simulink subsystem "wheelSlip"  (R2022b)
settings: Solver=VariableStepAuto  StartTime=0.0  StopTime=10.0  RelTol=1e-3
libraries: wheels x3
settings Model: Creator=serga  LastModifiedBy=serga

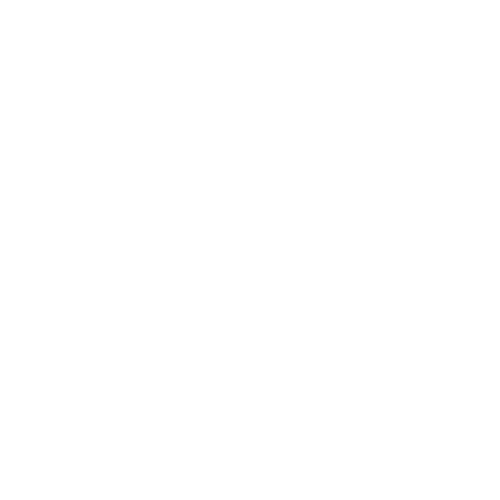
[thumbnail: Simulink's stored preview of the top-level diagram]
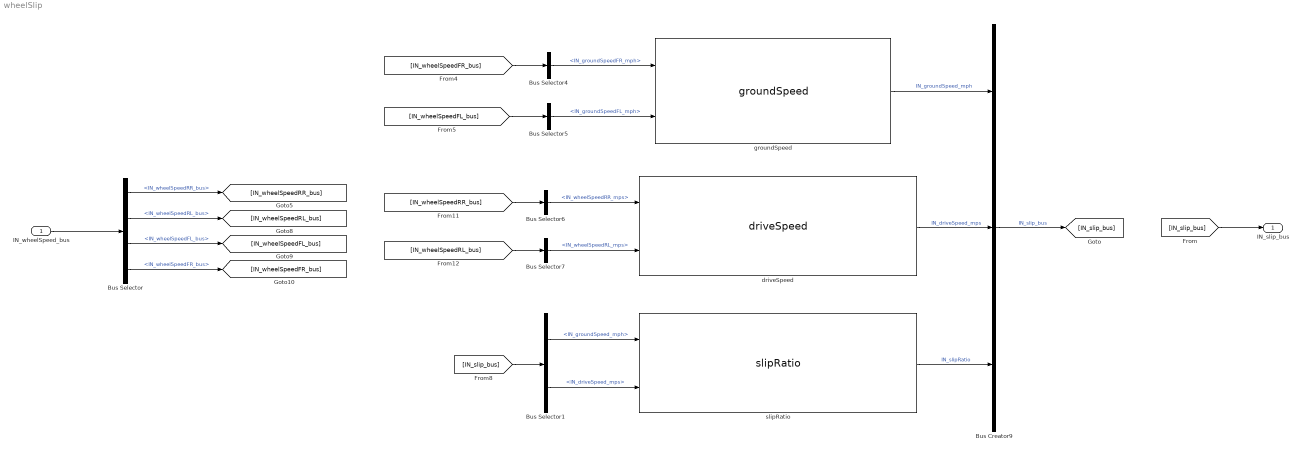
== system wheelSlip ==
  IN_wheelSpeed_bus : Inport
  Bus Creator9 : BusCreator  Inputs=3
  Bus Selector : BusSelector  OutputSignals=IN_wheelSpeedRR_bus,IN_wheelSpeedRL_bus,IN_wheelSpeedFL_bus,IN_wheelSpeedFR_bus
  Bus Selector1 : BusSelector  OutputSignals=IN_groundSpeed_mph,IN_driveSpeed_mps
  Bus Selector4 : BusSelector  OutputSignals=IN_groundSpeedFR_mph
  Bus Selector5 : BusSelector  OutputSignals=IN_groundSpeedFL_mph
  Bus Selector6 : BusSelector  OutputSignals=IN_wheelSpeedRR_mps
  Bus Selector7 : BusSelector  OutputSignals=IN_wheelSpeedRL_mps
  driveSpeed : wheels/driveSpeed  SystemSampleTime=-1  VariantActivationTime=update diagram  Latency=0  AutoFrameSizeCalculation=off
  groundSpeed : wheels/groundSpeed  SystemSampleTime=-1  VariantActivationTime=update diagram  Latency=0  AutoFrameSizeCalculation=off
  slipRatio : wheels/slipRatio  SystemSampleTime=-1  VariantActivationTime=update diagram  Latency=0  AutoFrameSizeCalculation=off
  IN_slip_bus : Outport
  wires:
  [IN_slip_bus] -> IN_slip_bus/1
  Bus Selector5/1 -> groundSpeed/2  "<IN_groundSpeedFL_mph>"
  [IN_wheelSpeedRR_bus] -> Bus Selector6/1
  [IN_wheelSpeedRL_bus] -> Bus Selector7/1
  Bus Selector4/1 -> groundSpeed/1  "<IN_groundSpeedFR_mph>"
  driveSpeed/1 -> Bus Creator9/2  "IN_driveSpeed_mps"
  [IN_wheelSpeedFR_bus] -> Bus Selector4/1
  IN_wheelSpeed_bus/1 -> Bus Selector/1
  [IN_wheelSpeedFL_bus] -> Bus Selector5/1
  Bus Selector/4 -> [IN_wheelSpeedFR_bus]  "<IN_wheelSpeedFR_bus>"
  Bus Selector/3 -> [IN_wheelSpeedFL_bus]  "<IN_wheelSpeedFL_bus>"
  Bus Creator9/1 -> [IN_slip_bus]  "IN_slip_bus"
  groundSpeed/1 -> Bus Creator9/1  "IN_groundSpeed_mph"
  Bus Selector/1 -> [IN_wheelSpeedRR_bus]  "<IN_wheelSpeedRR_bus>"
  Bus Selector7/1 -> driveSpeed/2  "<IN_wheelSpeedRL_mps>"
  [IN_slip_bus] -> Bus Selector1/1
  Bus Selector6/1 -> driveSpeed/1  "<IN_wheelSpeedRR_mps>"
  Bus Selector/2 -> [IN_wheelSpeedRL_bus]  "<IN_wheelSpeedRL_bus>"
  Bus Selector1/2 -> slipRatio/2  "<IN_driveSpeed_mps>"
  slipRatio/1 -> Bus Creator9/3  "IN_slipRatio"
  Bus Selector1/1 -> slipRatio/1  "<IN_groundSpeed_mph>"
